simulink model "hydrocracker"  (R2025a)
settings: Solver=VariableStepAuto  StartTime=0.0  StopTime=1000  RelTol=1e-3
values from neighbouring files (symbols this model uses):
  A = 5    [hydrocracking.m]
  alpha = 0.5    [hydrocracking.m]
  CH0 = 1000    [hydrocracking.m]
  CL0 = 0    [hydrocracking.m]
  CM0 = 0    [hydrocracking.m]
  dHrxn = -8e4    (= -80000)    [hydrocracking.m]
  Ea = 8e4    (= 80000)    [hydrocracking.m]
  F_H2in = 1    [hydrocracking.m]
  k0 = 1e6    (= 1000000)    [hydrocracking.m]
  nH2_0 = Pset * V_gas / (R*T0)    (= 2.00465078983)    [hydrocracking.m]
  Pset = 1e5    (= 100000)    [hydrocracking.m]
  R = 8.314    [hydrocracking.m]
  rhoCp = 4.0e6    (= 4000000)    [hydrocracking.m]
  T0 = 600    [hydrocracking.m]
  T_cool = 550    [hydrocracking.m]
  Tset = 600    [hydrocracking.m]
  U = 500    [hydrocracking.m]
  V_gas = 0.1    [hydrocracking.m]
  V_liq = 1.0    (= 1)    [hydrocracking.m]
libraries: slpidlib x2
settings Model: Creator=brown  LastModifiedBy=brown

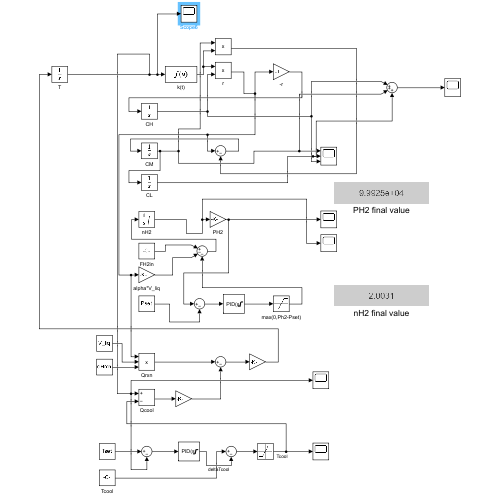
[thumbnail: Simulink's stored preview of the top-level diagram]
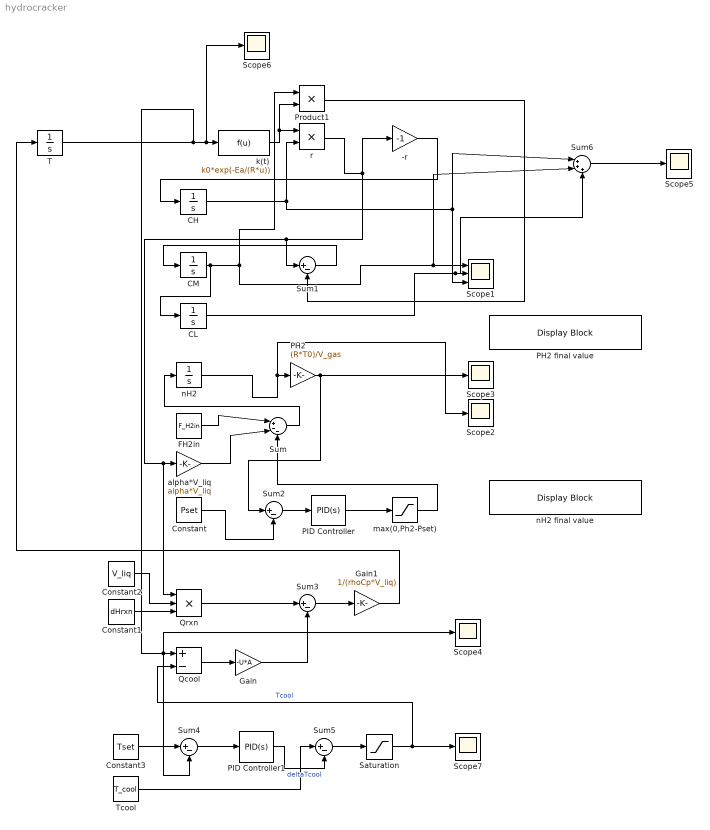
== system hydrocracker ==
  -r : Gain  Gain=-1
  CH : Integrator  InitialCondition=CH0
  CL : Integrator  InitialCondition=CL0
  CM : Integrator  InitialCondition=CM0
  Constant : Constant  Value=Pset
  Constant1 : Constant  Value=dHrxn
  Constant2 : Constant  Value=V_liq
  Constant3 : Constant  Value=Tset
  FH2in : Constant  Value=F_H2in
  Gain : Gain  Gain=-U*A
  Gain1 : Gain  Gain=1/(rhoCp*V_liq)
  PH2 : Gain  Gain=(R*T0)/V_gas
  PH2 final value : DisplayBlock  LabelPosition=Hide  Transparency=1  GridColor=[0.502, 0.502, 0.502]
  PID Controller : slpidlib/PID Controller  Controller=PID  Form=Parallel  TimeDomain=Continuous-time  UseExternalTs=off  SampleTime=-1  IntegratorMethod=Forward Euler  FilterMethod=Forward Euler  ControllerParametersSource=internal  P=5e-4  I=5e-5  UseKiTs=off  D=0  UseExternalDerivativeSource=off  N=100  UseFilter=on  TunerSelectOption=Transfer Function Based (PID Tuner App)  InitialConditionSource=internal  InitialConditionForIntegrator=0  InitialConditionForFilter=0  DifferentiatorICPrevScaledInput=0  ExternalReset=none  TrackingMode=off  Kt=1  LimitOutput=on  SatLimitsSource=internal  UpperSaturationLimit=inf  LowerSaturationLimit=0  LinearizeAsGain=on  AntiWindupMode=none  Kb=1  LimitIntegrator=off  UpperIntegratorSaturationLimit=inf  LowerIntegratorSaturationLimit=-inf  POutMin=[]  POutMax=[]  IOutMin=[]  IOutMax=[]  DOutMin=[]  DOutMax=[]  NOutMin=[]  NOutMax=[]  SumOutMin=[]  SumOutMax=[]  SaturationOutMin=[]  SaturationOutMax=[]  PParamMin=[]  PParamMax=[]  IParamMin=[]  IParamMax=[]  DParamMin=[]  DParamMax=[]  NParamMin=[]  NParamMax=[]  KbParamMin=[]  KbParamMax=[]  KtParamMin=[]  KtParamMax=[]  KbOutMin=[]  KbOutMax=[]  KtOutMin=[]  KtOutMax=[]  IntegratorOutMin=[]  IntegratorOutMax=[]  FilterOutMin=[]  FilterOutMax=[]  SumI1OutMin=[]  SumI1OutMax=[]  SumI2OutMin=[]  SumI2OutMax=[]  SumI3OutMin=[]  SumI3OutMax=[]  SumI4OutMin=[]  SumI4OutMax=[]  SumDOutMin=[]  SumDOutMax=[]  DifferentiatorOutMin=[]  DifferentiatorOutMax=[]  FilterDiffOutCoefMin=[]  FilterDiffOutCoefMax=[]  ReciprocalOutMin=[]  ReciprocalOutMax=[]  SumDenOutMin=[]  SumDenOutMax=[]  SumNumOutMin=[]  SumNumOutMax=[]  DivideOutMin=[]  DivideOutMax=[]  UdiffTsProdOutMin=[]  UdiffTsProdOutMax=[]  NTsProdOutMin=[]  NTsProdOutMax=[]  UintegralTsProdOutMin=[]  UintegralTsProdOutMax=[]  UngainTsProdOutMin=[]  UngainTsProdOutMax=[]  ClampingZeroOutDataTypeStr=Inherit: Inherit via back propagation  ClampingZeroOutMin=[]  ClampingZeroOutMax=[]  FilterDenConstantOutDataTypeStr=Inherit: Inherit via back propagation  FilterDenConstantOutMin=[]  FilterDenConstantOutMax=[]  PCopyOutDataTypeStr=Inherit: Inherit via back propagation  PCopyOutMin=[]  PCopyOutMax=[]  NCopyOutDataTypeStr=Inherit: Inherit via back propagation  NCopyOutMin=[]  NCopyOutMax=[]  IntegratorContinuousStateAttributes=''  IntegratorStateMustResolveToSignalObject=off  IntegratorRTWStateStorageClass=Auto  FilterContinuousStateAttributes=''  FilterStateMustResolveToSignalObject=off  FilterRTWStateStorageClass=Auto  ParallelPVariant=InternalParameters  IdealPVariant=Disabled  IVariant=InternalParameters  DVariant=InternalParameters  IntegratorVariant=Continuous  SatVariant=Enabled  AWVariant=Passthrough  PCopyVariant=Disabled  TRVariant=Disabled  FdbkBlocksVariant=Forward  IdealPFdbkVariant=Disabled  SatFdbkVariant=Disabled  DerivativeFilterVariant=ContFilter  NVariant=InternalParameters  NCopyVariant=Disabled  FilterICVariant=InternalICsFilter  IntegratorICVariant=InternalICs  ExternalResetVariant=Disabled  TRSumVariant=Passthrough  SumFdbkVariant=Disabled  SumVariant=Sum_PID  TsampFilterVariant=InternalTs  TsampNgainVariant=Passthrough  TsampIntegralVariant=Disabled_SignalSpec  ExternalSaturationOutDataTypeStr=Inherit: Same as second input  DerivativeSourceVariant=ErrorSignal  PreIntVariant=InternalPreInt
  PID Controller1 : slpidlib/PID Controller  Controller=PID  Form=Parallel  TimeDomain=Continuous-time  UseExternalTs=off  SampleTime=-1  IntegratorMethod=Forward Euler  FilterMethod=Forward Euler  ControllerParametersSource=internal  P=1.0  I=0.05  UseKiTs=off  D=0  UseExternalDerivativeSource=off  N=100  UseFilter=on  TunerSelectOption=Transfer Function Based (PID Tuner App)  InitialConditionSource=internal  InitialConditionForIntegrator=0  InitialConditionForFilter=0  DifferentiatorICPrevScaledInput=0  ExternalReset=none  TrackingMode=off  Kt=1  LimitOutput=on  SatLimitsSource=internal  UpperSaturationLimit=inf  LowerSaturationLimit=0  LinearizeAsGain=on  AntiWindupMode=none  Kb=1  LimitIntegrator=off  UpperIntegratorSaturationLimit=inf  LowerIntegratorSaturationLimit=-inf  POutMin=[]  POutMax=[]  IOutMin=[]  IOutMax=[]  DOutMin=[]  DOutMax=[]  NOutMin=[]  NOutMax=[]  SumOutMin=[]  SumOutMax=[]  SaturationOutMin=[]  SaturationOutMax=[]  PParamMin=[]  PParamMax=[]  IParamMin=[]  IParamMax=[]  DParamMin=[]  DParamMax=[]  NParamMin=[]  NParamMax=[]  KbParamMin=[]  KbParamMax=[]  KtParamMin=[]  KtParamMax=[]  KbOutMin=[]  KbOutMax=[]  KtOutMin=[]  KtOutMax=[]  IntegratorOutMin=[]  IntegratorOutMax=[]  FilterOutMin=[]  FilterOutMax=[]  SumI1OutMin=[]  SumI1OutMax=[]  SumI2OutMin=[]  SumI2OutMax=[]  SumI3OutMin=[]  SumI3OutMax=[]  SumI4OutMin=[]  SumI4OutMax=[]  SumDOutMin=[]  SumDOutMax=[]  DifferentiatorOutMin=[]  DifferentiatorOutMax=[]  FilterDiffOutCoefMin=[]  FilterDiffOutCoefMax=[]  ReciprocalOutMin=[]  ReciprocalOutMax=[]  SumDenOutMin=[]  SumDenOutMax=[]  SumNumOutMin=[]  SumNumOutMax=[]  DivideOutMin=[]  DivideOutMax=[]  UdiffTsProdOutMin=[]  UdiffTsProdOutMax=[]  NTsProdOutMin=[]  NTsProdOutMax=[]  UintegralTsProdOutMin=[]  UintegralTsProdOutMax=[]  UngainTsProdOutMin=[]  UngainTsProdOutMax=[]  ClampingZeroOutDataTypeStr=Inherit: Inherit via back propagation  ClampingZeroOutMin=[]  ClampingZeroOutMax=[]  FilterDenConstantOutDataTypeStr=Inherit: Inherit via back propagation  FilterDenConstantOutMin=[]  FilterDenConstantOutMax=[]  PCopyOutDataTypeStr=Inherit: Inherit via back propagation  PCopyOutMin=[]  PCopyOutMax=[]  NCopyOutDataTypeStr=Inherit: Inherit via back propagation  NCopyOutMin=[]  NCopyOutMax=[]  IntegratorContinuousStateAttributes=''  IntegratorStateMustResolveToSignalObject=off  IntegratorRTWStateStorageClass=Auto  FilterContinuousStateAttributes=''  FilterStateMustResolveToSignalObject=off  FilterRTWStateStorageClass=Auto  ParallelPVariant=InternalParameters  IdealPVariant=Disabled  IVariant=InternalParameters  DVariant=InternalParameters  IntegratorVariant=Continuous  SatVariant=Enabled  AWVariant=Passthrough  PCopyVariant=Disabled  TRVariant=Disabled  FdbkBlocksVariant=Forward  IdealPFdbkVariant=Disabled  SatFdbkVariant=Disabled  DerivativeFilterVariant=ContFilter  NVariant=InternalParameters  NCopyVariant=Disabled  FilterICVariant=InternalICsFilter  IntegratorICVariant=InternalICs  ExternalResetVariant=Disabled  TRSumVariant=Passthrough  SumFdbkVariant=Disabled  SumVariant=Sum_PID  TsampFilterVariant=InternalTs  TsampNgainVariant=Passthrough  TsampIntegralVariant=Disabled_SignalSpec  ExternalSaturationOutDataTypeStr=Inherit: Same as second input  DerivativeSourceVariant=ErrorSignal  PreIntVariant=InternalPreInt
  Product1 : Product
  Qcool : Sum  Inputs=+-
  Qrxn : Product  Inputs=3
  Saturation : Saturate  UpperLimit=600  LowerLimit=450
  Scope1 : Scope  NumInputPorts=3
      settings: ActiveDisplayYMinimum=-115.26738630932186  ActiveDisplayYMaximum=2026.48823667877
  Scope{2..7} (6 alike) : Scope
      Scope2 settings: ActiveDisplayYMinimum=-4.503216513253486  ActiveDisplayYMaximum=22.227202454879869  DataLoggingVariableName=ScopeData2
      Scope3 settings: ActiveDisplayYMinimum=-253622.65898233256  ActiveDisplayYMaximum=682252.73190292867  DataLoggingVariableName=ScopeData3
      Scope4 settings: ActiveDisplayYMinimum=575.73029004029047  ActiveDisplayYMaximum=606.60340044600207  DataLoggingVariableName=ScopeData4
      Scope5 settings: ActiveDisplayYMinimum=12051.812748407972  ActiveDisplayYMaximum=14909.091373153255  DataLoggingVariableName=ScopeData5
      Scope6 settings: ActiveDisplayYMinimum=376.16740458522753  ActiveDisplayYMaximum=766.51149347424075  DataLoggingVariableName=ScopeData6
      Scope7 settings: ActiveDisplayYMinimum=344.83039147979025  ActiveDisplayYMaximum=754.1193768014042  DataLoggingVariableName=ScopeData7
  Sum : Sum  Inputs=|+--
  Sum{1..5} (5 alike) : Sum  Inputs=|+-
  Sum6 : Sum  Inputs=|+++
  T : Integrator  InitialCondition=T0
  Tcool : Constant  Value=T_cool
  alpha*V_liq : Gain  Gain=alpha*V_liq
  k(t) : Fcn  Expr=k0*exp(-Ea/(R*u))
  max(0,Ph2-Pset) : Saturate  UpperLimit=inf  LowerLimit=0
  nH2 : Integrator  InitialCondition=nH2_0  LimitOutput=on  LowerSaturationLimit=0
  nH2 final value : DisplayBlock  LabelPosition=Hide  Transparency=1  GridColor=[0.502, 0.502, 0.502]
  r : Product
  wires:
  FH2in/1 -> Sum/1
  Sum1/1 -> CM/1
  nH2/1 -> PH2/1, Scope2/1
  CM/1 -> CL/1, Sum6/2, Scope1/1, Product1/1
  alpha*V_liq/1 -> Sum/2
  CH/1 -> Sum6/1, Scope1/3, r/2
  r/1 -> -r/1, Sum1/1, Qrxn/1, alpha*V_liq/1
  CL/1 -> Sum6/3, Scope1/2
  -r/1 -> CH/1
  PH2/1 -> Sum2/1, Scope3/1
  Product1/1 -> Sum1/2
  Sum/1 -> nH2/1
  T/1 -> Scope4/1, Qcool/1, Sum4/2, Scope6/1, k(t)/1
  k(t)/1 -> Product1/2, r/1
  Constant1/1 -> Qrxn/3
  Constant2/1 -> Qrxn/2
  Qcool/1 -> Gain/1
  Gain/1 -> Sum3/2
  Qrxn/1 -> Sum3/1
  Sum3/1 -> Gain1/1
  Gain1/1 -> T/1
  Sum2/1 -> PID Controller/1
  PID Controller/1 -> max(0,Ph2-Pset)/1
  max(0,Ph2-Pset)/1 -> Sum/3
  Constant/1 -> Sum2/2
  Constant3/1 -> Sum4/1
  Sum4/1 -> PID Controller1/1
  PID Controller1/1 -> Sum5/2  "deltaTcool"
  Sum5/1 -> Saturation/1
  Tcool/1 -> Sum5/1
  Saturation/1 -> Scope7/1, Qcool/2  "Tcool"
  Sum6/1 -> Scope5/1
